simulink model "Diagrama_Planta_todos_tanques"  (Simulink 8.0)
settings: Solver=ode45  StartTime=0.0  StopTime=10000  RelTol=1e-6
settings Model: Creator=pedro  LastModifiedBy=curso  ExtModeTrigMode=oneshot  ExtModeArmWhenConnect=off
settings DataIOCC: LimitDataPoints=off  SignalLoggingSaveFormat=ModelDataLogs  SaveOutput=off  SaveTime=off
settings OptimizationCC: BlockReduction=off  BooleanDataType=off
settings DebuggingCC: SaveWithParameterizedLinksMsg=none  SignalResolutionControl=TryResolveAllWithWarning  SolverPrmCheckMsg=none  MultiTaskDSMMsg=warning  MultiTaskCondExecSysMsg=none  FcnCallInpInsideContextMsg=UseLocalSettings  StrictBusMsg=None
settings HardwareCC: TargetUnknown=on
settings RTWCC: IncludeERTFirstTime=on
settings GRTTargetCC: CombineOutputUpdateFcns=off  GRTInterface=on

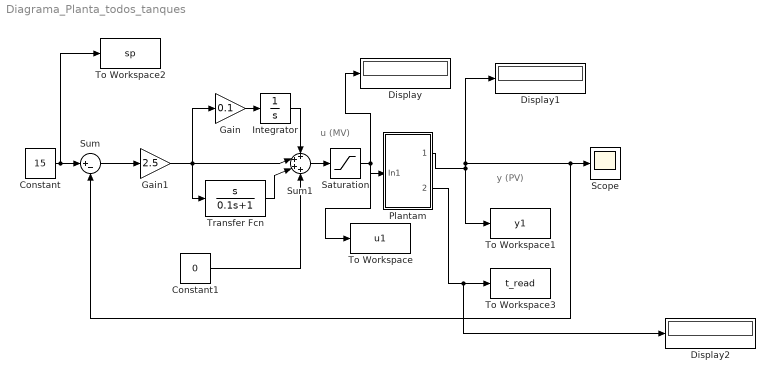
== system Diagrama_Planta_todos_tanques ==
  note: y (PV)
  note: u (MV)
  Constant : Constant  Value=15
  Constant1 : Constant  Value=0
  Display : Display
  Display1 : Display
  Display2 : Display
  Gain : Gain  Gain=0.1  SaturateOnIntegerOverflow=on  OutDataTypeStr=Inherit: Same as input  ParamDataTypeStr=Inherit: Same as input
  Gain1 : Gain  Gain=2.5  SaturateOnIntegerOverflow=on  OutDataTypeStr=Inherit: Same as input  ParamDataTypeStr=Inherit: Same as input
  Integrator : Integrator
  Plantam : Subsystem  mask{dt=1, machine='\\Laplace', server='Elipse.OPCSvr.1', tagout='Dados.Levels.Level_1.Value', tagin='IO_Module.AO_Pump.Pump_3.Value'}
      mask prompts: dt "Tempo de amostragem (s):"; machine "String com o nome do computador onde  está o servidor de OPC:"; server "String com o nome do servidor de OPC:"; tagout "String com o tag de saída  da planta (CV):"; tagin "String com o tag de entrada da planta (MV):"
      mask Display: image(imread('tanque','jpg'))
  Saturation : Saturate  UpperLimit=20  LowerLimit=4
  Scope : Scope
      settings: YMin=13  YMax=20
  Sum : Sum  Inputs=|+-  SaturateOnIntegerOverflow=on  InputSameDT=on  OutDataTypeStr=Inherit: Same as first input
  Sum1 : Sum  Inputs=++++  SaturateOnIntegerOverflow=on  InputSameDT=on  OutDataTypeStr=Inherit: Same as first input
  To Workspace : ToWorkspace  VariableName=u1  SampleTime=-1  SaveFormat=Structure With Time
  To Workspace1 : ToWorkspace  VariableName=y1  SampleTime=-1  SaveFormat=Structure With Time
  To Workspace2 : ToWorkspace  VariableName=sp  SampleTime=-1  SaveFormat=Structure With Time
  To Workspace3 : ToWorkspace  VariableName=t_read  SampleTime=-1  SaveFormat=Structure With Time
  Transfer Fcn : TransferFcn  Numerator=[1 0]  Denominator=[0.1 1]
  wires:
  Plantam/1(Out1) -> Display1/1, Scope/1, Sum/2, To Workspace1/1
  Constant/1 -> To Workspace2/1, Sum/1
  Gain/1 -> Integrator/1
  Integrator/1 -> Sum1/1
  Sum1/1 -> Saturation/1
  Saturation/1 -> Plantam/1(In1), To Workspace/1, Display/1
  Constant1/1 -> Sum1/4
  Sum/1 -> Gain1/1
  Gain1/1 -> Transfer Fcn/1, Gain/1, Sum1/2
  Transfer Fcn/1 -> Sum1/3
  Plantam/2(Out2) -> Display2/1, To Workspace3/1

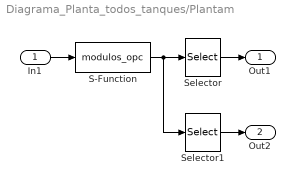
== system Diagrama_Planta_todos_tanques/Plantam ==
  In1 : Inport
  S-Function : S-Function  FunctionName=modulos_opc  Parameters=dt,machine,server,tagin,tagout  EnableBusSupport=off
  Selector : Selector  InputPortWidth=3  IndexOptions=Index vector (dialog)  Indices=[2]  OutputSizes=1
  Selector1 : Selector  InputPortWidth=3  IndexOptions=Index vector (dialog)  Indices=[3]  OutputSizes=1
  Out1 : Outport
  Out2 : Outport  Port=2
  wires:
  S-Function/1 -> Selector1/1, Selector/1
  Selector/1 -> Out1/1
  In1/1 -> S-Function/1
  Selector1/1 -> Out2/1
